simulink model "solar_collector_hot_water_tank_v1"  (R2017a)
settings: Solver=VariableStepAuto  StartTime=0.0  StopTime=50000  RelTol=1e-3
values from neighbouring files (symbols this model uses):
  a1 = Ac*eta/C_c    (= 0.000575964912281)    [Linearized_model.m]    (also in Linearized_model_v1.m; Maple_linearization.m = 0.000380952380952; solar_collector_init.m = 7.33988724098e-05)
  a2 = -U_L1*Ac/2/C_c    (= -0.00145487240829)    [Linearized_model.m]    (also in Linearized_model_v1.m = -0.00290974481659; Maple_linearization.m = 0.00111111111111; solar_collector_init.m = -0.000214080044529)
  a3 = -U_L2*Ac/C_c    (= -7.48006379585e-06)    [Linearized_model.m]    (also in Linearized_model_v1.m; Maple_linearization.m = -0.00222222222222; solar_collector_init.m = 0.000428160089057)
  a4 = V_c^-1    (= 333.333333333)    [Linearized_model.m]    (also in Linearized_model_v1.m; Maple_linearization.m = 666.666666667; solar_collector_init.m = 133.333333333)
  a5 = -a4    (= -333.333333333)    [Linearized_model.m]    (also in Linearized_model_v1.m; Maple_linearization.m = -666.666666667; solar_collector_init.m = -133.333333333)
  A_t = 0.5    [Linearized_model.m]    (also in Linearized_model_v1.m; Maple_linearization.m; solar_collector_init.m)
  C_ct = rho_c*c_c*V_ct    (= 326980.5)    [Maple_linearization.m]    (also in solar_collector_init.m)
  C_t = rho*c*V_s    (= 315000)    [Linearized_model.m]    (also in Linearized_model_v1.m; Maple_linearization.m = 3150000; solar_collector_init.m)
  U_t = 7    [Linearized_model.m]    (also in Linearized_model_v1.m = 250; Maple_linearization.m = 250; solar_collector_init.m = 250)
  V_ct = 0.075    [Linearized_model.m]    (also in Linearized_model_v1.m; Maple_linearization.m; solar_collector_init.m)
  V_t = 0.075    [Linearized_model.m]    (also in Linearized_model_v1.m; Maple_linearization.m = 0.75; solar_collector_init.m)
libraries: simulink x2
settings Model: Creator=info  LastModifiedBy=admin

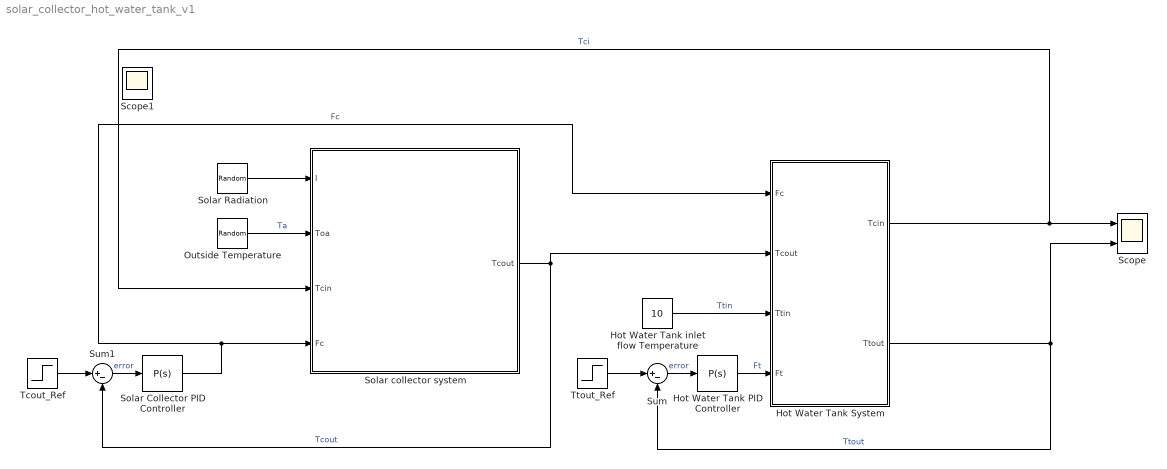
== system solar_collector_hot_water_tank_v1 ==
  Hot Water Tank PID Controller : simulink/Continuous/PID Controller  Controller=P  TimeDomain=Continuous-time  SampleTime=-1  IntegratorMethod=Forward Euler  FilterMethod=Forward Euler  Form=Parallel  UseFilter=on  ControllerParametersSource=internal  P=-0.0002*-1  I=1.2  D=0.01  N=100  InitialConditionSource=internal  InitialConditionForIntegrator=0  InitialConditionForFilter=0  ExternalReset=none  ZeroCross=off  LimitOutput=on  UpperSaturationLimit=0.0002  LowerSaturationLimit=0  LinearizeAsGain=on  AntiWindupMode=none  Kb=1  TrackingMode=off  Kt=1  PParamMin=[]  PParamMax=[]  IParamMin=[]  IParamMax=[]  DParamMin=[]  DParamMax=[]  NParamMin=[]  NParamMax=[]  KbParamMin=[]  KbParamMax=[]  KtParamMin=[]  KtParamMax=[]  POutMin=[]  POutMax=[]  IOutMin=[]  IOutMax=[]  DOutMin=[]  DOutMax=[]  NOutMin=[]  NOutMax=[]  KbOutMin=[]  KbOutMax=[]  KtOutMin=[]  KtOutMax=[]  IntegratorOutMin=[]  IntegratorOutMax=[]  FilterOutMin=[]  FilterOutMax=[]  SumOutMin=[]  SumOutMax=[]  SumI1OutMin=[]  SumI1OutMax=[]  SumI2OutMin=[]  SumI2OutMax=[]  SumI3OutMin=[]  SumI3OutMax=[]  SumDOutMin=[]  SumDOutMax=[]  SaturationOutMin=[]  SaturationOutMax=[]  IntegratorContinuousStateAttributes=''  IntegratorStateMustResolveToSignalObject=off  IntegratorRTWStateStorageClass=Auto  FilterContinuousStateAttributes=''  FilterStateMustResolveToSignalObject=off  FilterRTWStateStorageClass=Auto  DifferentiatorICPrevScaledInput=0  DifferentiatorOutMin=[]  DifferentiatorOutMax=[]  InitialConditionSetting=State (most efficient)
  Hot Water Tank System : Subsystem
      mask Display: image('hot_water_tank.PNG');
  Hot Water Tank inlet flow Temperature : Constant  Value=10
  Outside Temperature : RandomNumber  Mean=20  Variance=0.5  SampleTime=0.1
  Scope : Scope  NumInputPorts=2
  Solar Collector PID Controller : simulink/Continuous/PID Controller  Controller=P  TimeDomain=Continuous-time  SampleTime=-1  IntegratorMethod=Forward Euler  FilterMethod=Forward Euler  Form=Parallel  UseFilter=on  ControllerParametersSource=internal  P=0.002  I=1.2  D=0.01  N=100  InitialConditionSource=internal  InitialConditionForIntegrator=0  InitialConditionForFilter=0  ExternalReset=none  ZeroCross=off  LimitOutput=on  UpperSaturationLimit=0.00025  LowerSaturationLimit=0  LinearizeAsGain=on  AntiWindupMode=none  Kb=1  TrackingMode=off  Kt=1  PParamMin=[]  PParamMax=[]  IParamMin=[]  IParamMax=[]  DParamMin=[]  DParamMax=[]  NParamMin=[]  NParamMax=[]  KbParamMin=[]  KbParamMax=[]  KtParamMin=[]  KtParamMax=[]  POutMin=[]  POutMax=[]  IOutMin=[]  IOutMax=[]  DOutMin=[]  DOutMax=[]  NOutMin=[]  NOutMax=[]  KbOutMin=[]  KbOutMax=[]  KtOutMin=[]  KtOutMax=[]  IntegratorOutMin=[]  IntegratorOutMax=[]  FilterOutMin=[]  FilterOutMax=[]  SumOutMin=[]  SumOutMax=[]  SumI1OutMin=[]  SumI1OutMax=[]  SumI2OutMin=[]  SumI2OutMax=[]  SumI3OutMin=[]  SumI3OutMax=[]  SumDOutMin=[]  SumDOutMax=[]  SaturationOutMin=[]  SaturationOutMax=[]  IntegratorContinuousStateAttributes=''  IntegratorStateMustResolveToSignalObject=off  IntegratorRTWStateStorageClass=Auto  FilterContinuousStateAttributes=''  FilterStateMustResolveToSignalObject=off  FilterRTWStateStorageClass=Auto  DifferentiatorICPrevScaledInput=0  DifferentiatorOutMin=[]  DifferentiatorOutMax=[]  InitialConditionSetting=State (most efficient)
  Solar Radiation : RandomNumber  Mean=1000*1  Variance=0.5  SampleTime=0.1
  Solar collector system : Subsystem
      mask Display: image('collector_image.jpg');
  Sum : Sum  Inputs=|+-
  Sum1 : Sum  Inputs=|+-
  "Tcout_Ref " : Step  Time=20000  Before=60  After=60  SampleTime=0
  Ttout_Ref : Step  Time=30000  Before=47.5  After=47.5  SampleTime=0
  Scope1 : Scope
  wires:
  Hot Water Tank System/1("Tcin ") -> Solar collector system/3(Tcin), Scope/1  "Tci"
  Outside Temperature/1 -> Solar collector system/2(Toa)  "Ta"
  Solar Radiation/1 -> Solar collector system/1(I)
  Hot Water Tank System/2("Ttout ") -> Sum/2, Scope/2  "Ttout"
  Ttout_Ref/1 -> Sum/1
  Sum/1 -> Hot Water Tank PID Controller/1  "error"
  Solar Collector PID Controller/1 -> Hot Water Tank System/1("Fc "), Solar collector system/4(Fc)  "Fc"
  Hot Water Tank PID Controller/1 -> Hot Water Tank System/4(Ft)  "Ft"
  Hot Water Tank inlet flow Temperature/1 -> Hot Water Tank System/3("Ttin ")  "Ttin"
  Sum1/1 -> Solar Collector PID Controller/1  "error"
  "Tcout_Ref "/1 -> Sum1/1
  Solar collector system/1(Tcout) -> Sum1/2, Hot Water Tank System/2("Tcout ")  "Tcout"

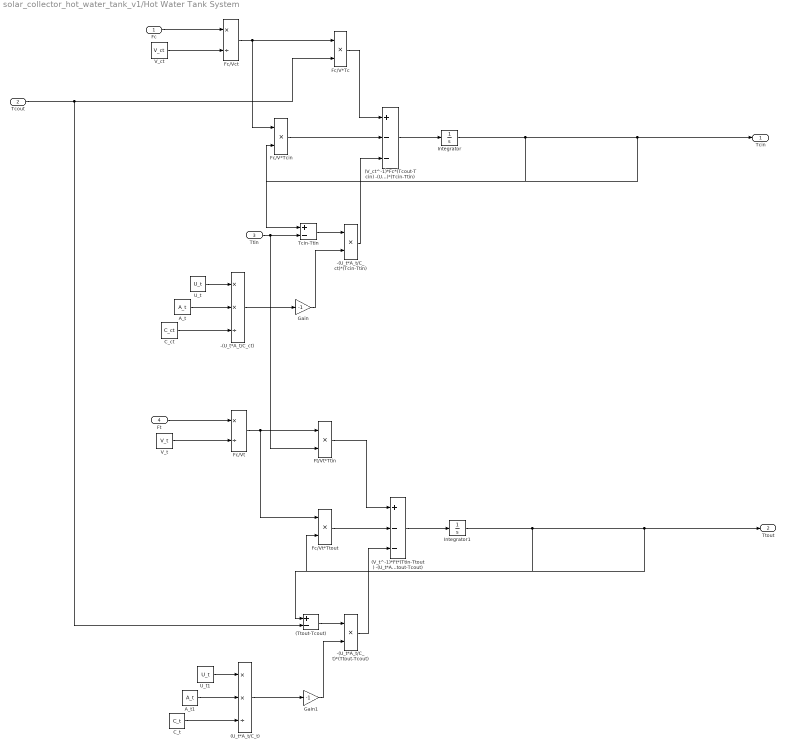
== system solar_collector_hot_water_tank_v1/Hot Water Tank System ==
  "Fc " : Inport
  "Tcout " : Inport  Port=2
  "Ttin " : Inport  Port=3
  Ft : Inport  Port=4
  (Ttout-Tcout) : Sum  Inputs=+-
  (U_t*A_t/C_t) : Product  Inputs=**/
  (V_ct^-1)*Fc*(Tcout-Tcin) -(U_t*A_t/C_ct)*(Tcin-Ttin) : Sum  Inputs=+--
  (V_t^-1)*Ft*(Ttin-Ttout) -(U_t*A_t/C_t)*(Ttout-Tcout) : Sum  Inputs=+--
  -(U_t*A_t/C_ct) : Product  Inputs=**/
  -(U_t*A_t/C_ct)*(Tcin-Ttin) : Product  Inputs=**
  -(U_t*A_t/C_t)*(Ttout-Tcout) : Product  Inputs=**
  A_t : Constant  Value=A_t
  A_t1 : Constant  Value=A_t
  "C_ct " : Constant  Value=C_ct
  C_t : Constant  Value=C_t
  Fc/V*Tc : Product  Inputs=**
  Fc/V*Tcin : Product  Inputs=**
  Fc/Vct : Product  Inputs=*/
  Fc/Vt : Product  Inputs=*/
  Fc/Vt*Ttout : Product  Inputs=**
  Ft/Vt*Ttin : Product  Inputs=**
  Gain : Gain  Gain=-1
  Gain1 : Gain  Gain=-1
  Integrator : Integrator  InitialCondition=16.87
  Integrator1 : Integrator  InitialCondition=16.87
  "Tcin-Ttin " : Sum  Inputs=+-
  U_t : Constant  Value=U_t
  U_t1 : Constant  Value=U_t
  "V_ct " : Constant  Value=V_ct
  V_t : Constant  Value=V_t
  "Tcin " : Outport
  "Ttout " : Outport  Port=2
  wires:
  "V_ct "/1 -> Fc/Vct/2
  "Fc "/1 -> Fc/Vct/1
  Fc/Vct/1 -> Fc/V*Tcin/1, Fc/V*Tc/1
  Integrator/1 -> Fc/V*Tcin/2, "Tcin "/1, "Tcin-Ttin "/1
  U_t/1 -> -(U_t*A_t/C_ct)/1
  "Tcout "/1 -> (Ttout-Tcout)/2, Fc/V*Tc/2
  A_t/1 -> -(U_t*A_t/C_ct)/2
  Fc/V*Tc/1 -> (V_ct^-1)*Fc*(Tcout-Tcin) -(U_t*A_t/C_ct)*(Tcin-Ttin)/1
  (V_ct^-1)*Fc*(Tcout-Tcin) -(U_t*A_t/C_ct)*(Tcin-Ttin)/1 -> Integrator/1
  -(U_t*A_t/C_ct)/1 -> Gain/1
  -(U_t*A_t/C_ct)*(Tcin-Ttin)/1 -> (V_ct^-1)*Fc*(Tcout-Tcin) -(U_t*A_t/C_ct)*(Tcin-Ttin)/3
  "Tcin-Ttin "/1 -> -(U_t*A_t/C_ct)*(Tcin-Ttin)/1
  Fc/V*Tcin/1 -> (V_ct^-1)*Fc*(Tcout-Tcin) -(U_t*A_t/C_ct)*(Tcin-Ttin)/2
  "C_ct "/1 -> -(U_t*A_t/C_ct)/3
  Gain/1 -> -(U_t*A_t/C_ct)*(Tcin-Ttin)/2
  (U_t*A_t/C_t)/1 -> Gain1/1
  V_t/1 -> Fc/Vt/2
  (Ttout-Tcout)/1 -> -(U_t*A_t/C_t)*(Ttout-Tcout)/1
  Integrator1/1 -> "Ttout "/1, Fc/Vt*Ttout/2, (Ttout-Tcout)/1
  Ft/Vt*Ttin/1 -> (V_t^-1)*Ft*(Ttin-Ttout) -(U_t*A_t/C_t)*(Ttout-Tcout)/1
  Fc/Vt/1 -> Fc/Vt*Ttout/1, Ft/Vt*Ttin/1
  A_t1/1 -> (U_t*A_t/C_t)/2
  Fc/Vt*Ttout/1 -> (V_t^-1)*Ft*(Ttin-Ttout) -(U_t*A_t/C_t)*(Ttout-Tcout)/2
  "Ttin "/1 -> Ft/Vt*Ttin/2, "Tcin-Ttin "/2
  (V_t^-1)*Ft*(Ttin-Ttout) -(U_t*A_t/C_t)*(Ttout-Tcout)/1 -> Integrator1/1
  -(U_t*A_t/C_t)*(Ttout-Tcout)/1 -> (V_t^-1)*Ft*(Ttin-Ttout) -(U_t*A_t/C_t)*(Ttout-Tcout)/3
  Ft/1 -> Fc/Vt/1
  U_t1/1 -> (U_t*A_t/C_t)/1
  C_t/1 -> (U_t*A_t/C_t)/3
  Gain1/1 -> -(U_t*A_t/C_t)*(Ttout-Tcout)/2

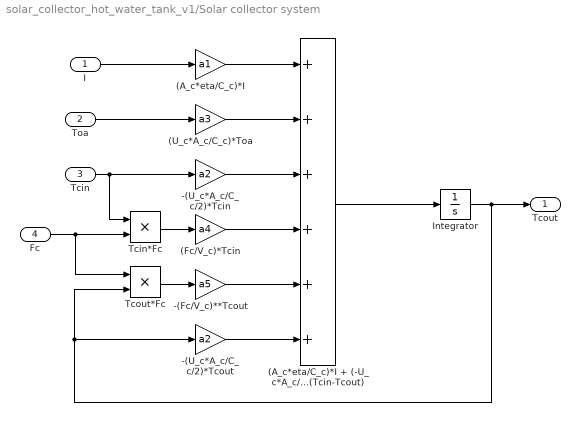
== system solar_collector_hot_water_tank_v1/Solar collector system ==
  I : Inport
  Toa : Inport  Port=2
  Tcin : Inport  Port=3
  Fc : Inport  Port=4
  (A_c*eta/C_c)*I : Gain  Gain=a1
  (A_c*eta/C_c)*I + (-U_c*A_c/C_c)*((Tcin+Tcout)/2-Toa) + Fc/V_c*(Tcin-Tcout) : Sum  Inputs=++++++
  (Fc/V_c)*Tcin : Gain  Gain=a4
  (U_c*A_c/C_c)*Toa : Gain  Gain=a3
  "-(Fc/V_c)**Tcout " : Gain  Gain=a5
  -(U_c*A_c/C_c/2)*Tcin : Gain  Gain=a2
  "-(U_c*A_c/C_c/2)*Tcout " : Gain  Gain=a2
  Integrator : Integrator  InitialCondition=10
  Tcin*Fc : Product  Inputs=**
  Tcout*Fc : Product  Inputs=**
  Tcout : Outport
  wires:
  I/1 -> (A_c*eta/C_c)*I/1
  Integrator/1 -> "-(U_c*A_c/C_c/2)*Tcout "/1, Tcout*Fc/2, Tcout/1
  (A_c*eta/C_c)*I + (-U_c*A_c/C_c)*((Tcin+Tcout)/2-Toa) + Fc/V_c*(Tcin-Tcout)/1 -> Integrator/1
  Fc/1 -> Tcout*Fc/1, Tcin*Fc/2
  (A_c*eta/C_c)*I/1 -> (A_c*eta/C_c)*I + (-U_c*A_c/C_c)*((Tcin+Tcout)/2-Toa) + Fc/V_c*(Tcin-Tcout)/1
  Toa/1 -> (U_c*A_c/C_c)*Toa/1
  Tcin/1 -> Tcin*Fc/1, -(U_c*A_c/C_c/2)*Tcin/1
  (U_c*A_c/C_c)*Toa/1 -> (A_c*eta/C_c)*I + (-U_c*A_c/C_c)*((Tcin+Tcout)/2-Toa) + Fc/V_c*(Tcin-Tcout)/2
  -(U_c*A_c/C_c/2)*Tcin/1 -> (A_c*eta/C_c)*I + (-U_c*A_c/C_c)*((Tcin+Tcout)/2-Toa) + Fc/V_c*(Tcin-Tcout)/3
  "-(Fc/V_c)**Tcout "/1 -> (A_c*eta/C_c)*I + (-U_c*A_c/C_c)*((Tcin+Tcout)/2-Toa) + Fc/V_c*(Tcin-Tcout)/5
  Tcin*Fc/1 -> (Fc/V_c)*Tcin/1
  (Fc/V_c)*Tcin/1 -> (A_c*eta/C_c)*I + (-U_c*A_c/C_c)*((Tcin+Tcout)/2-Toa) + Fc/V_c*(Tcin-Tcout)/4
  Tcout*Fc/1 -> "-(Fc/V_c)**Tcout "/1
  "-(U_c*A_c/C_c/2)*Tcout "/1 -> (A_c*eta/C_c)*I + (-U_c*A_c/C_c)*((Tcin+Tcout)/2-Toa) + Fc/V_c*(Tcin-Tcout)/6
